simulink model "servoController"  (R2015a)
settings: Solver=ode45  StartTime=0.0  StopTime=10.0  RelTol=1e-3
libraries: cstblocks x3
settings Model: Creator=kavindu  LastModifiedBy=kavindu

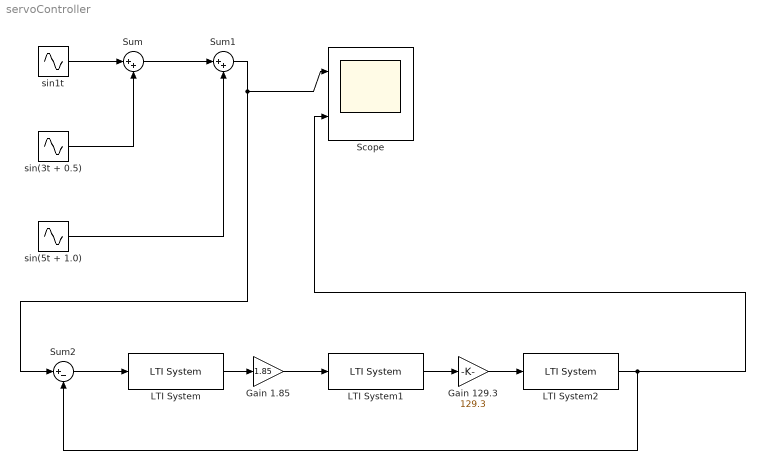
== system servoController ==
  Gain 1.85 : Gain  Gain=1.85
  Gain 129.3 : Gain  Gain=129.3
  LTI System : cstblocks/LTI System  sys=tf([1 0.95],[1 0.1])  IC=[]
  LTI System1 : cstblocks/LTI System  sys=tf([1 10.8],[1 37])  IC=[]
  LTI System2 : cstblocks/LTI System  sys=tf([1 3],[1 7 32 80])  IC=[]
  Scope : Scope  NumInputPorts=2
      settings: YMin=-5~-5  YMax=5~5
  Sum : Sum  Inputs=|++
  Sum1 : Sum  Inputs=|++
  Sum2 : Sum  Inputs=|+-
  sin(3t + 0.5) : Sin  Frequency=3  Phase=0.5  SampleTime=0
  sin(5t + 1.0) : Sin  Frequency=5  Phase=1.0  SampleTime=0
  sin1t : Sin  SampleTime=0
  wires:
  sin1t/1 -> Sum/1
  sin(3t + 0.5)/1 -> Sum/2
  Sum/1 -> Sum1/1
  sin(5t + 1.0)/1 -> Sum1/2
  LTI System/1 -> Gain 1.85/1
  LTI System1/1 -> Gain 129.3/1
  Gain 129.3/1 -> LTI System2/1
  Sum1/1 -> Sum2/1, Scope/1
  Gain 1.85/1 -> LTI System1/1
  LTI System2/1 -> Scope/2, Sum2/2
  Sum2/1 -> LTI System/1
